simulink model "foc_caller_test"  (R2024a)
settings: Solver=FixedStepAuto  StartTime=0.0  StopTime=0.02  FixedStep=5e-5  RelTol=1e-3
settings Model: Creator=黄钟锐  LastModifiedBy=黄钟锐
settings SFSimCC: SimCustomHeaderCode="#include \"sim/foc_sim.h\""
settings SFSimCC: SimUserSources=|
  | src\sim\foc_sim.c
  | src\control\current_controller.c
  | src\foc\foc_math.c
  | src\foc\svpwm.c
settings SFSimCC: SimUserIncludeDirs=|
  | include
  | src
  | src\sim
  | src\control
  | src\foc

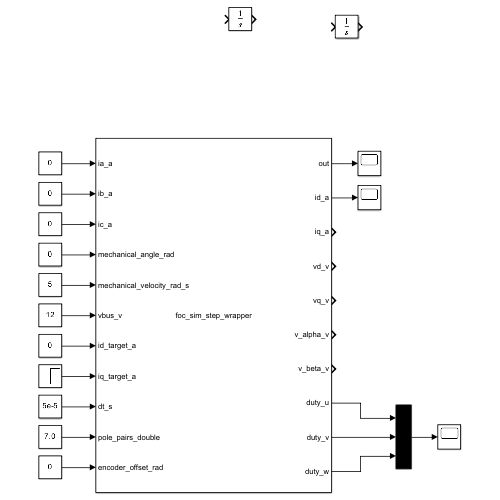
[thumbnail: Simulink's stored preview of the top-level diagram]
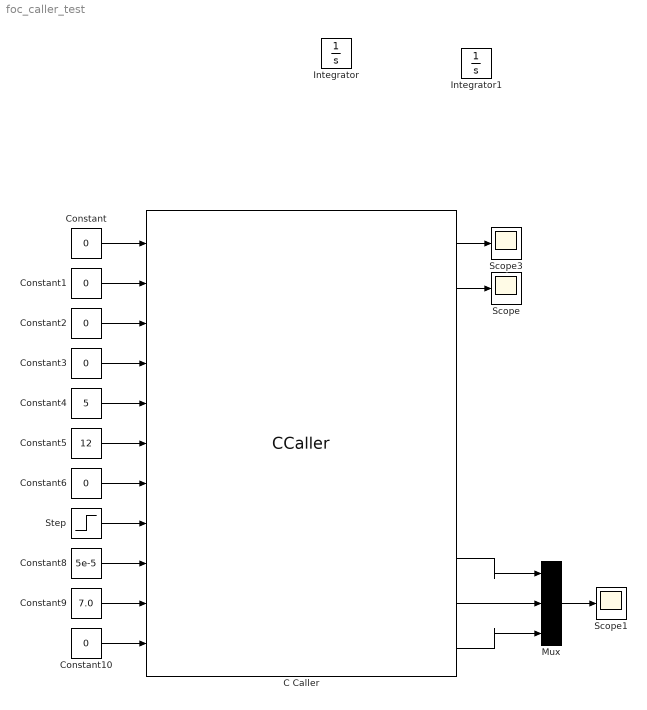
== system foc_caller_test ==
  C Caller : CCaller  FunctionName=foc_sim_step_wrapper  PortSpecificationStruct="%)30     .    &\"0   8    (     @         %    \"    !4    !     0         %  0 \"0    $    _    07)G3F%M90  4&]R=$YA;64 4V-O<&4     26YD97@     5'EP90      4VEZ90      27-';&]B86P   X    P    !@    @    $          4    (     0    ,    !         !   P!O=70 #@   #     &    \"     0         !0    @    !     P    $         $  # &]U=  .    .     8    (    !          %    \"     $    &     0         0  ...(+12085 chars)"  SampleTime=5e-5
  Constant{,1..3,6,10} (6 alike) : Constant  Value=0
  Constant4 : Constant  Value=5
  Constant5 : Constant  Value=12
  Constant8 : Constant  Value=5e-5
  Constant9 : Constant  Value=7.0
  Integrator : Integrator
  Integrator1 : Integrator
  Mux : Mux  Inputs=3
  Scope : Scope
  Scope1 : Scope
  Scope3 : Scope
  Step : Step  Time=0.005  After=0.5  SampleTime=5e-5
  wires:
  Constant/1 -> C Caller/1
  Constant1/1 -> C Caller/2
  Constant2/1 -> C Caller/3
  Constant3/1 -> C Caller/4
  Constant4/1 -> C Caller/5
  Constant5/1 -> C Caller/6
  Constant6/1 -> C Caller/7
  Step/1 -> C Caller/8
  Constant8/1 -> C Caller/9
  Constant9/1 -> C Caller/10
  Constant10/1 -> C Caller/11
  C Caller/2 -> Scope/1
  C Caller/8 -> Mux/1
  C Caller/9 -> Mux/2
  C Caller/10 -> Mux/3
  C Caller/1 -> Scope3/1
  Mux/1 -> Scope1/1
